simulink model "high_speed_passenger_train"  (R2018a)
settings: Solver=ode15s  StartTime=0.0  StopTime=180  RelTol=1e-7
libraries: simulink_extras x1
settings Model: Creator=dstep12  LastModifiedBy=dstep12
settings SolverCC: MaxOrder=2  MaxConsecutiveMinStep=10  SolverResetMethod=Robust
settings DataIOCC: Refine=10

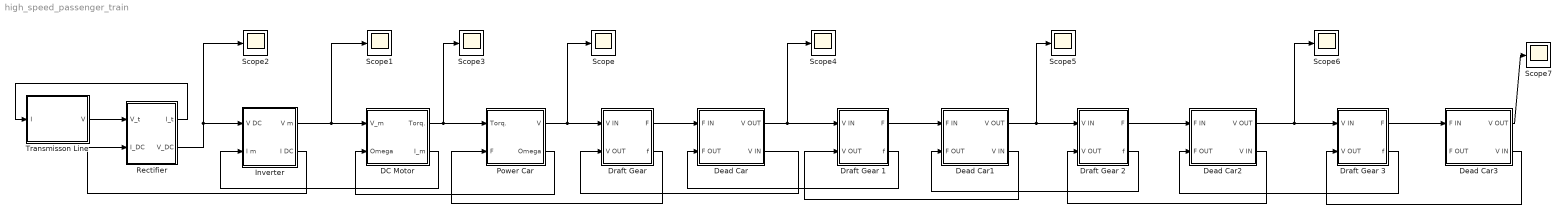
== system high_speed_passenger_train ==
  "DC Motor " : Subsystem
  Dead Car : Subsystem
  Dead Car1 : Subsystem
  Dead Car2 : Subsystem
  Dead Car3 : Subsystem
  "Draft Gear " : Subsystem
  Draft Gear 1 : Subsystem
  Draft Gear 2 : Subsystem
  Draft Gear 3 : Subsystem
  Inverter : Subsystem
  "Power Car " : Subsystem
  "Rectifier " : Subsystem
  Scope{,1..7} (8 alike) : Scope
  Transmisson Line : Subsystem
  wires:
  Inverter/1(V m) -> "DC Motor "/1("V_m "), Scope1/1
  Transmisson Line/1(V) -> "Rectifier "/1(V_t)
  Inverter/2("I DC ") -> "Rectifier "/2(I_DC)
  "Rectifier "/1("I_t ") -> Transmisson Line/1(I)
  "Rectifier "/2(V_DC) -> Inverter/1("V DC "), Scope2/1
  "DC Motor "/2("I_m ") -> Inverter/2(I m)
  "DC Motor "/1(Torq.) -> "Power Car "/1(Torq.), Scope3/1
  "Power Car "/2("Omega ") -> "DC Motor "/2("Omega ")
  "Power Car "/1("V ") -> "Draft Gear "/1("V IN "), Scope/1
  Dead Car/1(V OUT) -> Draft Gear 1/1("V IN "), Scope4/1
  "Draft Gear "/1("F ") -> Dead Car/1(F IN)
  "Draft Gear "/2(f) -> "Power Car "/2(F)
  Dead Car/2("V IN ") -> "Draft Gear "/2("V OUT ")
  Draft Gear 1/2(f) -> Dead Car/2(F OUT)
  Draft Gear 1/1("F ") -> Dead Car1/1(F IN)
  Dead Car1/2("V IN ") -> Draft Gear 1/2("V OUT ")
  Dead Car1/1(V OUT) -> Scope5/1, Draft Gear 2/1("V IN ")
  Draft Gear 2/1("F ") -> Dead Car2/1(F IN)
  Dead Car2/1(V OUT) -> Scope6/1, Draft Gear 3/1("V IN ")
  Draft Gear 3/1("F ") -> Dead Car3/1(F IN)
  Draft Gear 2/2(f) -> Dead Car1/2(F OUT)
  Dead Car2/2("V IN ") -> Draft Gear 2/2("V OUT ")
  Draft Gear 3/2(f) -> Dead Car2/2(F OUT)
  Dead Car3/2("V IN ") -> Draft Gear 3/2("V OUT ")
  Dead Car3/1(V OUT) -> Scope7/1

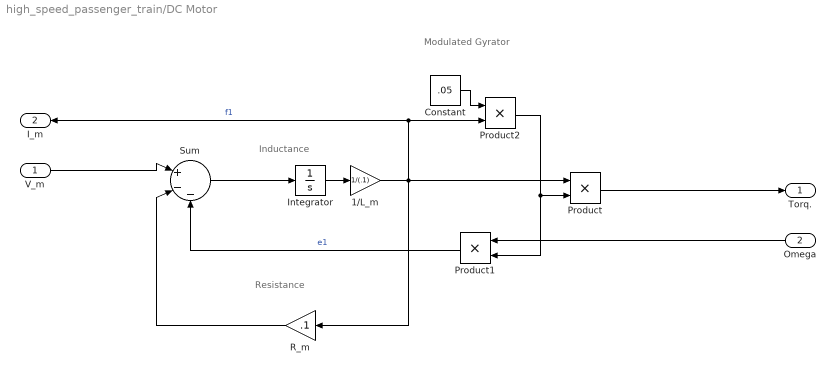
== system high_speed_passenger_train/DC Motor  ==
  note: Modulated Gyrator
  note: Inductance
  note: Resistance
  "V_m " : Inport
  "Omega " : Inport  Port=2
  1/L_m : Gain  Gain=1/(.1)
  Constant : Constant  Value=.05
  Integrator : Integrator
  Product : Product
  Product1 : Product
  Product2 : Product
  R_m : Gain  Gain=.1
  Sum : Sum  Inputs=|+--
  Torq. : Outport
  "I_m " : Outport  Port=2
  wires:
  Integrator/1 -> 1/L_m/1
  "Omega "/1 -> Product1/1
  Sum/1 -> Integrator/1
  Product/1 -> Torq./1
  1/L_m/1 -> Product2/2, "I_m "/1, R_m/1, Product/1  "f1"
  Constant/1 -> Product2/1
  Product1/1 -> Sum/3  "e1"
  R_m/1 -> Sum/2
  Product2/1 -> Product1/2, Product/2
  "V_m "/1 -> Sum/1

== system high_speed_passenger_train/Dead Car ==
  F IN : Inport
  F OUT : Inport  Port=2
  Gain : Gain  Gain=1/80000
  Integrator : Integrator
  Sum : Sum  Inputs=|-+
  V OUT : Outport
  "V IN " : Outport  Port=2
  wires:
  Sum/1 -> Integrator/1
  F IN/1 -> Sum/2
  Gain/1 -> V OUT/1, "V IN "/1
  F OUT/1 -> Sum/1
  Integrator/1 -> Gain/1

== system high_speed_passenger_train/Dead Car1 ==
  F IN : Inport
  F OUT : Inport  Port=2
  Gain : Gain  Gain=1/80000
  Integrator : Integrator
  Sum : Sum  Inputs=|-+
  V OUT : Outport
  "V IN " : Outport  Port=2
  wires:
  Sum/1 -> Integrator/1
  F IN/1 -> Sum/2
  Gain/1 -> V OUT/1, "V IN "/1
  F OUT/1 -> Sum/1
  Integrator/1 -> Gain/1

== system high_speed_passenger_train/Dead Car2 ==
  F IN : Inport
  F OUT : Inport  Port=2
  Gain : Gain  Gain=1/80000
  Integrator : Integrator
  Sum : Sum  Inputs=|-+
  V OUT : Outport
  "V IN " : Outport  Port=2
  wires:
  Sum/1 -> Integrator/1
  F IN/1 -> Sum/2
  Gain/1 -> V OUT/1, "V IN "/1
  F OUT/1 -> Sum/1
  Integrator/1 -> Gain/1

== system high_speed_passenger_train/Dead Car3 ==
  F IN : Inport
  F OUT : Inport  Port=2
  Gain : Gain  Gain=1/80000
  Integrator : Integrator
  Sum : Sum  Inputs=|-+
  V OUT : Outport
  "V IN " : Outport  Port=2
  wires:
  Sum/1 -> Integrator/1
  F IN/1 -> Sum/2
  Gain/1 -> V OUT/1, "V IN "/1
  F OUT/1 -> Sum/1
  Integrator/1 -> Gain/1

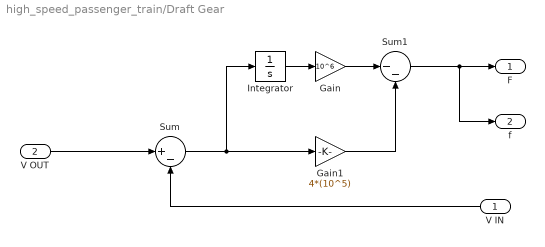
== system high_speed_passenger_train/Draft Gear  ==
  "V IN " : Inport
  "V OUT " : Inport  Port=2
  Gain : Gain  Gain=10^6
  Gain1 : Gain  Gain=4*(10^5)
  Integrator : Integrator
  Sum : Sum  Inputs=|+-
  Sum1 : Sum  Inputs=|--
  "F " : Outport
  f : Outport  Port=2
  wires:
  Gain/1 -> Sum1/1
  "V OUT "/1 -> Sum/1
  Gain1/1 -> Sum1/2
  Sum/1 -> Integrator/1, Gain1/1
  Integrator/1 -> Gain/1
  "V IN "/1 -> Sum/2
  Sum1/1 -> f/1, "F "/1

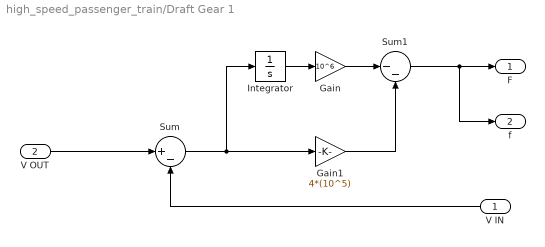
== system high_speed_passenger_train/Draft Gear 1 ==
  "V IN " : Inport
  "V OUT " : Inport  Port=2
  Gain : Gain  Gain=10^6
  Gain1 : Gain  Gain=4*(10^5)
  Integrator : Integrator
  Sum : Sum  Inputs=|+-
  Sum1 : Sum  Inputs=|--
  "F " : Outport
  f : Outport  Port=2
  wires:
  Gain/1 -> Sum1/1
  "V OUT "/1 -> Sum/1
  Gain1/1 -> Sum1/2
  Sum/1 -> Integrator/1, Gain1/1
  Integrator/1 -> Gain/1
  "V IN "/1 -> Sum/2
  Sum1/1 -> f/1, "F "/1

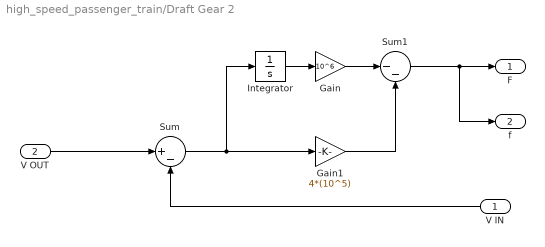
== system high_speed_passenger_train/Draft Gear 2 ==
  "V IN " : Inport
  "V OUT " : Inport  Port=2
  Gain : Gain  Gain=10^6
  Gain1 : Gain  Gain=4*(10^5)
  Integrator : Integrator
  Sum : Sum  Inputs=|+-
  Sum1 : Sum  Inputs=|--
  "F " : Outport
  f : Outport  Port=2
  wires:
  Gain/1 -> Sum1/1
  "V OUT "/1 -> Sum/1
  Gain1/1 -> Sum1/2
  Sum/1 -> Integrator/1, Gain1/1
  Integrator/1 -> Gain/1
  "V IN "/1 -> Sum/2
  Sum1/1 -> f/1, "F "/1

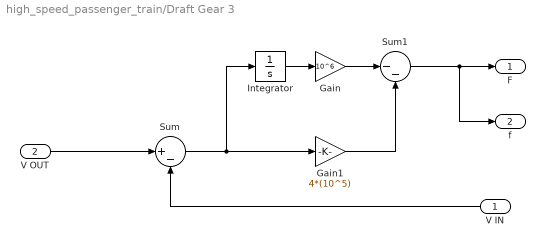
== system high_speed_passenger_train/Draft Gear 3 ==
  "V IN " : Inport
  "V OUT " : Inport  Port=2
  Gain : Gain  Gain=10^6
  Gain1 : Gain  Gain=4*(10^5)
  Integrator : Integrator
  Sum : Sum  Inputs=|+-
  Sum1 : Sum  Inputs=|--
  "F " : Outport
  f : Outport  Port=2
  wires:
  Gain/1 -> Sum1/1
  "V OUT "/1 -> Sum/1
  Gain1/1 -> Sum1/2
  Sum/1 -> Integrator/1, Gain1/1
  Integrator/1 -> Gain/1
  "V IN "/1 -> Sum/2
  Sum1/1 -> f/1, "F "/1

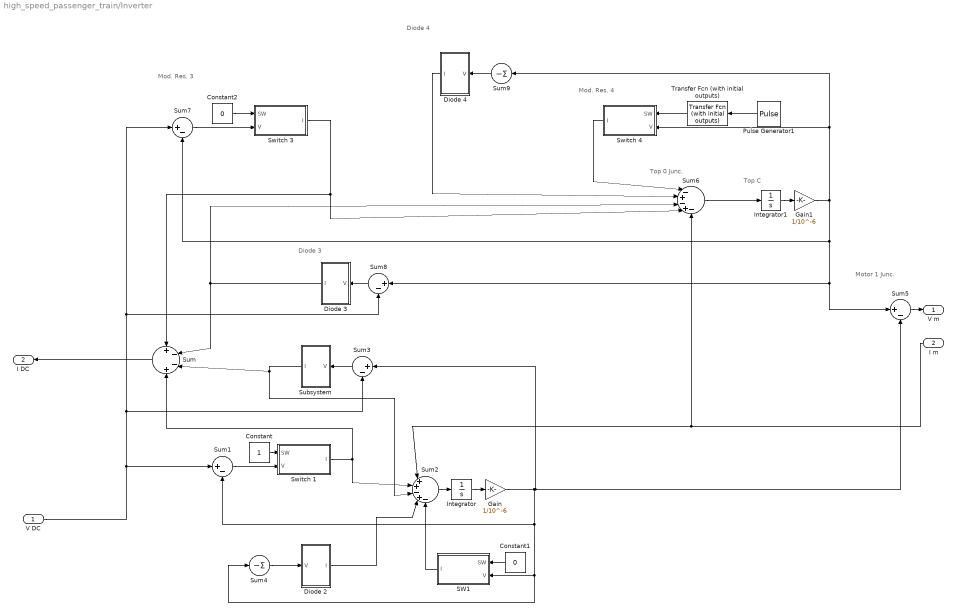
== system high_speed_passenger_train/Inverter ==
  note: Diode 3
  note: Mod. Res. 3
  note: Mod. Res. 4
  note: Diode 4
  note: Top 0 Junc.
  note: Top C
  note: Motor 1 Junc.
  "V DC " : Inport
  I m : Inport  Port=2
  Constant : Constant
  Constant1 : Constant  Value=0
  Constant2 : Constant  Value=0
  Diode 2 : Subsystem
  Diode 3 : Subsystem
  Diode 4 : Subsystem
  Gain : Gain  Gain=1/10^-6
  Gain1 : Gain  Gain=1/10^-6
  Integrator : Integrator
  Integrator1 : Integrator
  Pulse Generator1 : DiscretePulseGenerator  PulseType=Time based  Period=0.02  PulseWidth=50
  SW1 : Subsystem
  Subsystem : Subsystem
  Sum : Sum  Inputs=+--+
  Sum{1,3,5,7..8} (5 alike) : Sum  Inputs=|+-
  Sum2 : Sum  Inputs=|++-+-
  Sum4 : Sum  Inputs=-
  Sum6 : Sum  Inputs=|-+-+-
  Sum9 : Sum  Inputs=-
  Switch 1 : Subsystem
  Switch 3 : Subsystem
  "Switch 4 " : Subsystem
  Transfer Fcn (with initial outputs) : simulink_extras/Additional Linear/Transfer Fcn (with initial outputs)  N=[1/1e-4]  D="[1  1/1e-4]"  Y0=0  U0=0
  V m : Outport
  "I DC " : Outport  Port=2
  wires:
  Subsystem/1(I) -> Sum2/3, Sum/3
  I m/1 -> Sum2/1, Sum6/5
  Sum5/1 -> V m/1
  SW1/1(I) -> Sum2/5
  Transfer Fcn (with initial outputs)/1 -> "Switch 4 "/1(SW)
  Sum3/1 -> Subsystem/1(V)
  "Switch 4 "/1(I) -> Sum6/1
  Gain/1 -> Sum1/2, Sum4/1, SW1/2(V), Sum5/2, Sum3/1
  Sum7/1 -> Switch 3/2(V)
  Switch 1/1(I) -> Sum2/2, Sum/4
  Gain1/1 -> Sum9/1, "Switch 4 "/2(V), Sum8/1, Sum5/1, Sum7/2
  Sum1/1 -> Switch 1/2(V)
  Sum4/1 -> Diode 2/1(V)
  Sum6/1 -> Integrator1/1
  "V DC "/1 -> Sum7/1, Sum8/2, Sum3/2, Sum1/1
  Diode 2/1(I) -> Sum2/4
  Sum2/1 -> Integrator/1
  Diode 4/1(I) -> Sum6/2
  Sum9/1 -> Diode 4/1(V)
  Switch 3/1(I) -> Sum6/4, Sum/1
  Integrator/1 -> Gain/1
  Pulse Generator1/1 -> Transfer Fcn (with initial outputs)/1
  Diode 3/1(I) -> Sum/2, Sum6/3
  Constant2/1 -> Switch 3/1(SW)
  Sum8/1 -> Diode 3/1(V)
  Constant/1 -> Switch 1/1(SW)
  Integrator1/1 -> Gain1/1
  Sum/1 -> "I DC "/1
  Constant1/1 -> SW1/1(SW)

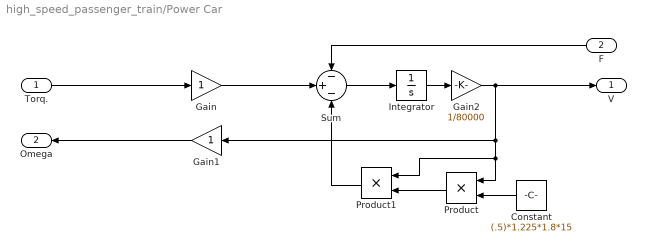
== system high_speed_passenger_train/Power Car  ==
  Torq. : Inport
  F : Inport  Port=2
  Constant : Constant  Value=(.5)*1.225*1.8*15
  Gain : Gain
  Gain1 : Gain
  Gain2 : Gain  Gain=1/80000
  Integrator : Integrator
  Product : Product
  Product1 : Product
  Sum : Sum  Inputs=-+-
  "V " : Outport
  "Omega " : Outport  Port=2
  wires:
  Sum/1 -> Integrator/1
  F/1 -> Sum/1
  Constant/1 -> Product/2
  Integrator/1 -> Gain2/1
  Gain/1 -> Sum/2
  Product1/1 -> Sum/3
  Gain2/1 -> "V "/1, Gain1/1, Product1/1, Product/1
  Product/1 -> Product1/2
  Gain1/1 -> "Omega "/1
  Torq./1 -> Gain/1

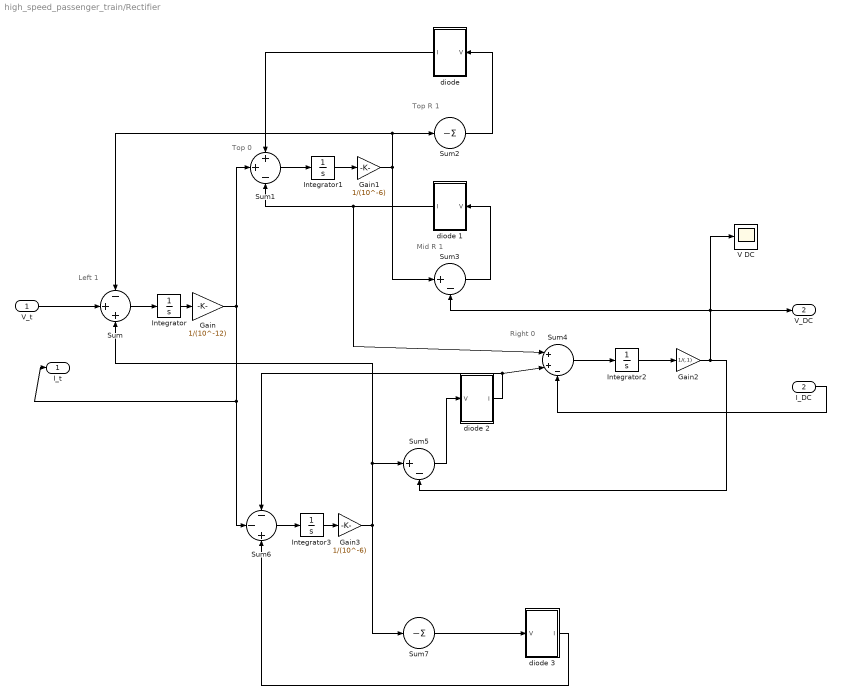
== system high_speed_passenger_train/Rectifier  ==
  note: Right 0
  note: Mid R 1
  note: Top R 1
  note: Left 1
  note: Top 0
  V_t : Inport
  I_DC : Inport  Port=2
  Gain : Gain  Gain=1/(10^-12)
  Gain1 : Gain  Gain=1/(10^-6)
  Gain2 : Gain  Gain=1/(.1)
  Gain3 : Gain  Gain=1/(10^-6)
  Integrator{,1..3} (4 alike) : Integrator
  Sum : Sum  Inputs=-++
  Sum1 : Sum  Inputs=++-
  Sum2 : Sum  Inputs=-
  Sum3 : Sum  Inputs=|+-
  Sum4 : Sum  Inputs=|++-
  Sum5 : Sum  Inputs=|+-
  Sum6 : Sum  Inputs=--+
  Sum7 : Sum  Inputs=-
  "V DC " : Scope
  "diode " : Subsystem
  diode 1 : Subsystem
  diode 2 : Subsystem
  diode 3 : Subsystem
  "I_t " : Outport
  V_DC : Outport  Port=2
  wires:
  diode 3/1(I) -> Sum6/3
  Gain1/1 -> Sum3/1, Sum/1, Sum2/1
  Integrator1/1 -> Gain1/1
  Sum4/1 -> Integrator2/1
  Gain3/1 -> Sum7/1, Sum/3, Sum5/1
  Gain/1 -> "I_t "/1, Sum6/2, Sum1/2
  Gain2/1 -> Sum5/2, V_DC/1, "V DC "/1, Sum3/2
  "diode "/1(I) -> Sum1/1
  V_t/1 -> Sum/2
  diode 1/1(I) -> Sum4/1, Sum1/3
  Integrator/1 -> Gain/1
  Sum1/1 -> Integrator1/1
  Sum2/1 -> "diode "/1(V)
  diode 2/1(I) -> Sum4/2, Sum6/1
  Sum3/1 -> diode 1/1(V)
  Sum7/1 -> diode 3/1(V)
  Integrator2/1 -> Gain2/1
  Sum/1 -> Integrator/1
  Sum6/1 -> Integrator3/1
  Integrator3/1 -> Gain3/1
  Sum5/1 -> diode 2/1(V)
  I_DC/1 -> Sum4/3

== system high_speed_passenger_train/Transmisson Line ==
  I : Inport
  Gain : Gain  Gain=10
  Pant. Res : Gain  Gain=.025
  Sine Wave : Sin  Amplitude=25000*sqrt(2)  Frequency=100*pi  SampleTime=0
  Sum : Sum  Inputs=|+-
  Trans. : Gain  Gain=1/10
  V : Outport
  wires:
  Trans./1 -> V/1
  Gain/1 -> Pant. Res/1
  I/1 -> Gain/1
  Sum/1 -> Trans./1
  Pant. Res/1 -> Sum/2
  Sine Wave/1 -> Sum/1

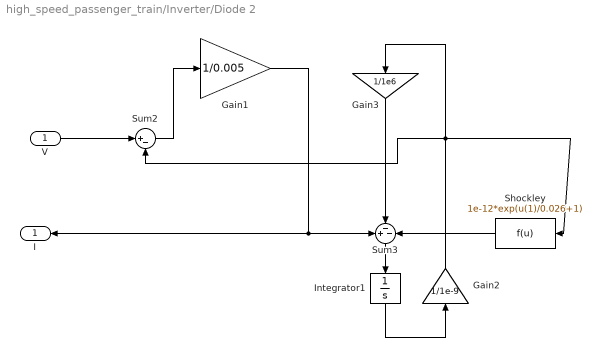
== system high_speed_passenger_train/Inverter/Diode 2 ==
  V : Inport
  Gain1 : Gain  Gain=1/0.005
  Gain2 : Gain  Gain=1/1e-9
  Gain3 : Gain  Gain=1/1e6
  Integrator1 : Integrator  AbsoluteTolerance=1e-12
  Shockley : Fcn  Expr=1e-12*exp(u(1)/0.026+1)
  Sum2 : Sum  Inputs=|+-
  Sum3 : Sum  Inputs=+--
  I : Outport
  wires:
  Gain3/1 -> Sum3/2
  Gain2/1 -> Sum2/2, Shockley/1, Gain3/1
  Sum2/1 -> Gain1/1
  Sum3/1 -> Integrator1/1
  Gain1/1 -> I/1, Sum3/1
  Shockley/1 -> Sum3/3
  Integrator1/1 -> Gain2/1
  V/1 -> Sum2/1

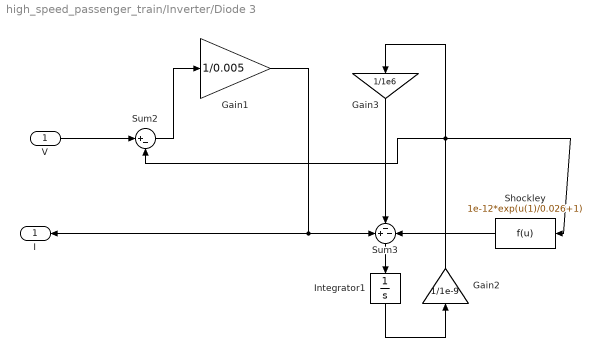
== system high_speed_passenger_train/Inverter/Diode 3 ==
  V : Inport
  Gain1 : Gain  Gain=1/0.005
  Gain2 : Gain  Gain=1/1e-9
  Gain3 : Gain  Gain=1/1e6
  Integrator1 : Integrator  AbsoluteTolerance=1e-12
  Shockley : Fcn  Expr=1e-12*exp(u(1)/0.026+1)
  Sum2 : Sum  Inputs=|+-
  Sum3 : Sum  Inputs=+--
  I : Outport
  wires:
  Gain3/1 -> Sum3/2
  Gain2/1 -> Sum2/2, Shockley/1, Gain3/1
  Sum2/1 -> Gain1/1
  Sum3/1 -> Integrator1/1
  Gain1/1 -> I/1, Sum3/1
  Shockley/1 -> Sum3/3
  Integrator1/1 -> Gain2/1
  V/1 -> Sum2/1

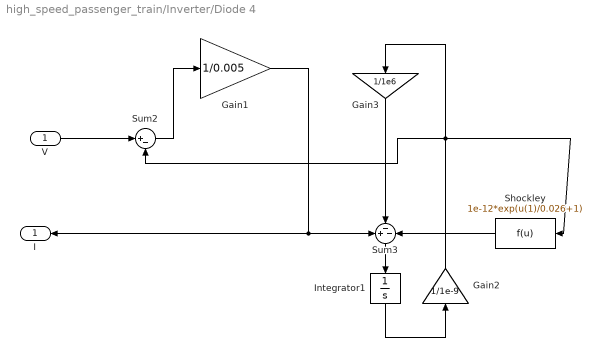
== system high_speed_passenger_train/Inverter/Diode 4 ==
  V : Inport
  Gain1 : Gain  Gain=1/0.005
  Gain2 : Gain  Gain=1/1e-9
  Gain3 : Gain  Gain=1/1e6
  Integrator1 : Integrator  AbsoluteTolerance=1e-12
  Shockley : Fcn  Expr=1e-12*exp(u(1)/0.026+1)
  Sum2 : Sum  Inputs=|+-
  Sum3 : Sum  Inputs=+--
  I : Outport
  wires:
  Gain3/1 -> Sum3/2
  Gain2/1 -> Sum2/2, Shockley/1, Gain3/1
  Sum2/1 -> Gain1/1
  Sum3/1 -> Integrator1/1
  Gain1/1 -> I/1, Sum3/1
  Shockley/1 -> Sum3/3
  Integrator1/1 -> Gain2/1
  V/1 -> Sum2/1

== system high_speed_passenger_train/Inverter/SW1 ==
  SW : Inport
  V : Inport  Port=2
  Constant1 : Constant  Value=1/0.001
  Constant2 : Constant  Value=1/10e6
  Product : Product
  Product1 : Product
  Sum : Sum  Inputs=|+-
  Sum1 : Sum  Inputs=++|
  I : Outport
  wires:
  V/1 -> Product/2
  Product/1 -> I/1
  Constant1/1 -> Sum/1
  SW/1 -> Product1/2
  Sum1/1 -> Product/1
  Constant2/1 -> Sum1/1, Sum/2
  Sum/1 -> Product1/1
  Product1/1 -> Sum1/2

== system high_speed_passenger_train/Inverter/Subsystem ==
  V : Inport
  Gain1 : Gain  Gain=1/0.005
  Gain2 : Gain  Gain=1/1e-9
  Gain3 : Gain  Gain=1/1e6
  Integrator1 : Integrator  AbsoluteTolerance=1e-12
  Shockley : Fcn  Expr=1e-12*exp(u(1)/0.026+1)
  Sum2 : Sum  Inputs=|+-
  Sum3 : Sum  Inputs=+--
  I : Outport
  wires:
  Gain3/1 -> Sum3/2
  Gain2/1 -> Sum2/2, Shockley/1, Gain3/1
  Sum2/1 -> Gain1/1
  Sum3/1 -> Integrator1/1
  Gain1/1 -> I/1, Sum3/1
  Shockley/1 -> Sum3/3
  Integrator1/1 -> Gain2/1
  V/1 -> Sum2/1

== system high_speed_passenger_train/Inverter/Switch 1 ==
  SW : Inport
  V : Inport  Port=2
  Constant1 : Constant  Value=1/0.001
  Constant2 : Constant  Value=1/10e6
  Product : Product
  Product1 : Product
  Sum : Sum  Inputs=|+-
  Sum1 : Sum  Inputs=++|
  I : Outport
  wires:
  V/1 -> Product/2
  Product/1 -> I/1
  Constant1/1 -> Sum/1
  SW/1 -> Product1/2
  Sum1/1 -> Product/1
  Constant2/1 -> Sum1/1, Sum/2
  Sum/1 -> Product1/1
  Product1/1 -> Sum1/2

== system high_speed_passenger_train/Inverter/Switch 3 ==
  SW : Inport
  V : Inport  Port=2
  Constant1 : Constant  Value=1/0.001
  Constant2 : Constant  Value=1/10e6
  Product : Product
  Product1 : Product
  Sum : Sum  Inputs=|+-
  Sum1 : Sum  Inputs=++|
  I : Outport
  wires:
  V/1 -> Product/2
  Product/1 -> I/1
  Constant1/1 -> Sum/1
  SW/1 -> Product1/2
  Sum1/1 -> Product/1
  Constant2/1 -> Sum1/1, Sum/2
  Sum/1 -> Product1/1
  Product1/1 -> Sum1/2

== system high_speed_passenger_train/Inverter/Switch 4  ==
  SW : Inport
  V : Inport  Port=2
  Constant1 : Constant  Value=1/0.001
  Constant2 : Constant  Value=1/10e6
  Product : Product
  Product1 : Product
  Sum : Sum  Inputs=|+-
  Sum1 : Sum  Inputs=++|
  I : Outport
  wires:
  V/1 -> Product/2
  Product/1 -> I/1
  Constant1/1 -> Sum/1
  SW/1 -> Product1/2
  Sum1/1 -> Product/1
  Constant2/1 -> Sum1/1, Sum/2
  Sum/1 -> Product1/1
  Product1/1 -> Sum1/2

== system high_speed_passenger_train/Rectifier /diode  ==
  V : Inport
  Gain2 : Gain  Gain=1/0.005
  Gain3 : Gain  Gain=1/1e-9
  Gain4 : Gain  Gain=1/1e6
  Integrator2 : Integrator  AbsoluteTolerance=1e-12
  Shockley : Fcn  Expr=1e-12*exp(u(1)/0.026+1)
  Sum4 : Sum  Inputs=|+-
  Sum5 : Sum  Inputs=+--
  I : Outport
  wires:
  Gain2/1 -> I/1, Sum5/1
  Sum4/1 -> Gain2/1
  Shockley/1 -> Sum5/3
  Sum5/1 -> Integrator2/1
  Integrator2/1 -> Gain3/1
  Gain3/1 -> Sum4/2, Shockley/1, Gain4/1
  Gain4/1 -> Sum5/2
  V/1 -> Sum4/1

== system high_speed_passenger_train/Rectifier /diode 1 ==
  V : Inport
  Gain2 : Gain  Gain=1/0.005
  Gain3 : Gain  Gain=1/1e-9
  Gain4 : Gain  Gain=1/1e6
  Integrator2 : Integrator  AbsoluteTolerance=1e-12
  Shockley : Fcn  Expr=1e-12*exp(u(1)/0.026+1)
  Sum4 : Sum  Inputs=|+-
  Sum5 : Sum  Inputs=+--
  I : Outport
  wires:
  Gain2/1 -> I/1, Sum5/1
  Sum4/1 -> Gain2/1
  Shockley/1 -> Sum5/3
  Sum5/1 -> Integrator2/1
  Integrator2/1 -> Gain3/1
  Gain3/1 -> Sum4/2, Shockley/1, Gain4/1
  Gain4/1 -> Sum5/2
  V/1 -> Sum4/1

== system high_speed_passenger_train/Rectifier /diode 2 ==
  V : Inport
  Gain2 : Gain  Gain=1/0.005
  Gain3 : Gain  Gain=1/1e-9
  Gain4 : Gain  Gain=1/1e6
  Integrator2 : Integrator  AbsoluteTolerance=1e-12
  Shockley : Fcn  Expr=1e-12*exp(u(1)/0.026+1)
  Sum4 : Sum  Inputs=|+-
  Sum5 : Sum  Inputs=+--
  I : Outport
  wires:
  Gain2/1 -> I/1, Sum5/1
  Sum4/1 -> Gain2/1
  Shockley/1 -> Sum5/3
  Sum5/1 -> Integrator2/1
  Integrator2/1 -> Gain3/1
  Gain3/1 -> Sum4/2, Shockley/1, Gain4/1
  Gain4/1 -> Sum5/2
  V/1 -> Sum4/1

== system high_speed_passenger_train/Rectifier /diode 3 ==
  V : Inport
  Gain2 : Gain  Gain=1/0.005
  Gain3 : Gain  Gain=1/1e-9
  Gain4 : Gain  Gain=1/1e6
  Integrator2 : Integrator  AbsoluteTolerance=1e-12
  Shockley : Fcn  Expr=1e-12*exp(u(1)/0.026+1)
  Sum4 : Sum  Inputs=|+-
  Sum5 : Sum  Inputs=+--
  I : Outport
  wires:
  Gain2/1 -> I/1, Sum5/1
  Sum4/1 -> Gain2/1
  Shockley/1 -> Sum5/3
  Sum5/1 -> Integrator2/1
  Integrator2/1 -> Gain3/1
  Gain3/1 -> Sum4/2, Shockley/1, Gain4/1
  Gain4/1 -> Sum5/2
  V/1 -> Sum4/1
